simulink model "Yanwen_of_controller_mode"  (R2020a)
settings: Solver=FixedStepAuto  StartTime=0.0  StopTime=inf  FixedStep=SAMPLE_TIME  RelTol=1e-3
undefined symbols (not defined in the file or in its folder): D_saturation, DiscIntNeverNeededParam, G_correct_gain, GEAR_RATIO, I_saturation, MAX_QD, MAX_QDD, MAX_TAU, MJ_Test1_torque_mode, N, N_PLoop, N_VLoop, NUM_SEGMS, P_Kp, P_saturation, q_zero_offset, SAMPLE_TIME, theta_max, theta_min, v_des_saturation, V_Kd, V_Ki, V_Kp, v_threshold_I_stop
libraries: ighEthercatLib x38, simulink x9, simulink_extras x8, dspstat3 x3
(part 1 of 2)
settings Model: ExplicitPartitioning=on  Creator=86166  LastModifiedBy=win
settings OptimizationCC: EnhancedBackFolding=on  PassReuseOutputArgsThreshold=0  OptimizeBlockOrder=speed  DifferentSizesBufferReuse=on  OptimizationCustomize=off
settings DebuggingCC: ParameterTunabilityLossMsg=error
settings HardwareCC: ProdBitPerLong=64  ProdHWDeviceType=Intel->x86-64 (Linux 64)  TargetBitPerPointer=64  TargetBitPerSizeT=64  TargetBitPerPtrDiffT=64  TargetLongLongMode=on  TargetIntDivRoundTo=Zero  TargetEndianess=LittleEndian  TargetWordSize=64  TargetHWDeviceType=Custom Processor->MATLAB Host Computer  ProdEqTarget=off
settings RTWCC: Description=Generic Real-Time Target  SystemTargetFile=links_rtlnx_grt.tlc  GenCodeOnly=on  TemplateMakefile=links_rtlnx_grt.tmf  GenerateReport=on  RTWVerbose=off  CustomLibrary=libethercat.a  LaunchReport=on
settings CodeAppCC: ForceParamTrailComments=on  OperatorAnnotations=on
settings STFCustomTargetCC: ModelReferenceCompliant=off  CombineOutputUpdateFcns=on  SystemTargetFile=links_rtlnx_grt.tlc
settings GRTTargetCC: TargetLangStandard=C89/C90 (ANSI)  ModelReferenceCompliant=off  ParMdlRefBuildCompliant=off  CompOptLevelCompliant=off  ConcurrentExecutionCompliant=off  MatFileLogging=off  CPPClassGenCompliant=off  UseToolchainInfoCompliant=off  RTWCAPISignals=on  RTWCAPIParams=on  RTWCAPIRootIO=on

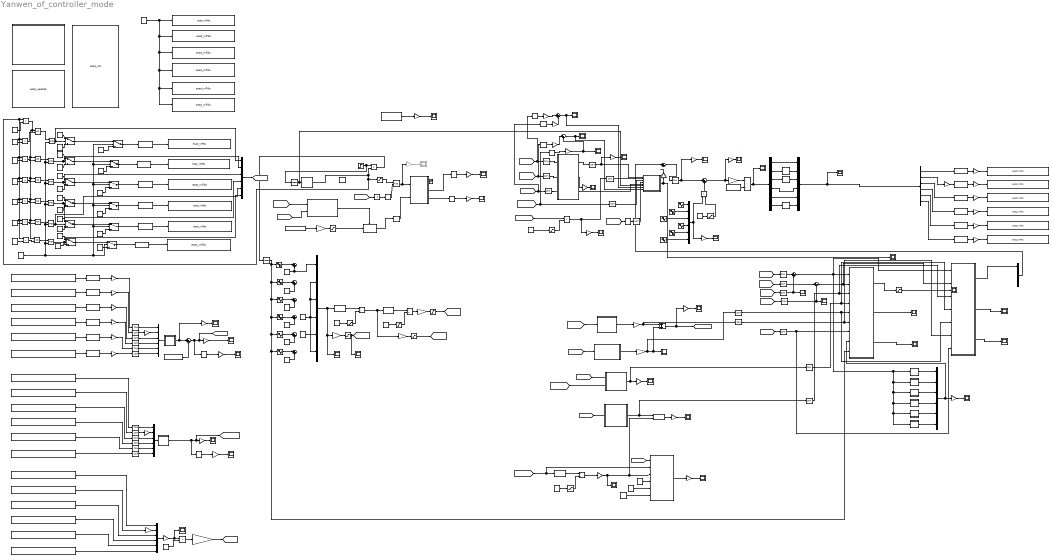
== system Yanwen_of_controller_mode ==
  note: 嵌套双环控制模块
  note: 8是位置模式，9是速度模式，10是力矩模式
  note: 关节使能之后才能启动轨迹规划
  note: 轨迹规划模块
  note: 编码器零位偏移量
  note: 模型识别变量模块
  note: 15是使能，6是去使能，128是驱动器初始化
  note: 连杆端的力矩值
  note: 使能控制
  note: 动力学模型计算模块
  note: 当前速度为零并且回到初始位置才能更新目标点
  note: 如果做数值仿真，则将阶跃信号替换sim_Step
  note: 模型初始化配置
  note: tau是连杆端力矩N.m，电机力矩输入单位是mN.m
  note: 所有的角度计算是基于弧度rad
  note: 滤波要用
  1dof_controller : MATLAB Function  TreatAsAtomicUnit=on
  Add2 : Sum
  C : Scope
  C_tau : Gain
  Compare To Zero : simulink/Logic and Bit Operations/Compare To Zero  relop=>  OutDataTypeStr=boolean
  Constant : Constant  Value=10
  Constant1 : Constant  Value=SAMPLE_TIME  SampleTime=SAMPLE_TIME
  Constant10 : Constant  Value=MJ_Test1_torque_mode
  Constant11 : Constant  Value=0
  Constant{12..13,17..21} (7 alike) : Constant  Value=6
  Constant{14..16,22..24} (6 alike) : Constant  Value=15
  Constant2 : Constant  Value=SAMPLE_TIME  SampleTime=SAMPLE_TIME
  Constant25 : Constant  Value=86  SampleTime=-1
  Constant26 : Constant  Value=4  SampleTime=-1
  Constant27 : Constant  Value=-5
  Constant28 : Constant  Value=10
  Constant29 : Constant  Value=0
  Constant3 : Constant  Value=0.001
  Constant30 : Constant  Value=90
  Constant33 : Constant  Value=SAMPLE_TIME  SampleTime=SAMPLE_TIME
  Constant{4..9} (6 alike) : Constant  Value=128
  Data Type Conversion{1,3..7,13..17,19} (12 alike) : DataTypeConversion  OutDataTypeStr=double
  Data Type Conversion{2,8..12} (6 alike) : DataTypeConversion  OutDataTypeStr=int32
  Demux : Demux  Outputs=6
  Demux2 : Demux  Outputs=6
  Difference : simulink/Discrete/Difference  ICPrevInput=zeros(1,6)  OutMin=[]  OutMax=[]  OutDataType=fixdt(1, 16)  OutScaling=2^-10  DoSatur=off
  Difference1 : simulink/Discrete/Difference  ICPrevInput=zeros(1,6)  OutMin=[]  OutMax=[]  OutDataType=fixdt(1, 16)  OutScaling=2^-10  DoSatur=off
  Difference2 : simulink/Discrete/Difference  ICPrevInput=zeros(1,6)  OutMin=[]  OutMax=[]  OutDataType=fixdt(1, 16)  OutScaling=2^-10  DoSatur=off
  Discrete-Time Integrator : DiscreteIntegrator  SampleTime=-1  ICPrevOutput=DiscIntNeverNeededParam  ICPrevScaledInput=DiscIntNeverNeededParam
  Discrete-Time Integrator1 : DiscreteIntegrator  SampleTime=-1  ICPrevOutput=DiscIntNeverNeededParam  ICPrevScaledInput=DiscIntNeverNeededParam
  Divide : Product  Inputs=*/  OutDataTypeStr=double
  Divide1 : Product  Inputs=*/
  Divide2 : Product  Inputs=*/
  Divide3 : Product  Inputs=*/
  Enabled Subsystem1 : Subsystem  TreatAsAtomicUnit=on
  G : Scope
  G_and_fric : Gain
  G_correct_gain : Gain  Gain=G_correct_gain
  Gain : Gain
  Gain{10..14,16} (6 alike) : Gain  OutDataTypeStr=Inherit: Same as input  ParamDataTypeStr=Inherit: Same as input
  JOINT2 Average1 : dspstat3/Moving Average  Method=Sliding window  ForgettingFactorPort=off  SpecifyWindowLength=on  WindowLength=2  ForgettingFactor=0.9  SimulateUsing=Code generation
  JOINT3 Average : dspstat3/Moving Average  Method=Sliding window  ForgettingFactorPort=off  SpecifyWindowLength=on  WindowLength=2  ForgettingFactor=0.9  SimulateUsing=Code generation
  JOINT3 Average1 : dspstat3/Moving Average  Method=Sliding window  ForgettingFactorPort=off  SpecifyWindowLength=on  WindowLength=3  ForgettingFactor=0.9  SimulateUsing=Code generation
  Kff_coef : Constant
  Logical Operator{,1..5} (6 alike) : Logic  Operator=OR  AllPortsSameDT=off  OutDataTypeStr=boolean
  Logical Operator{6..12} (7 alike) : Logic  AllPortsSameDT=off  OutDataTypeStr=boolean
  Logical Operator13 : Logic  Operator=NOT  AllPortsSameDT=off  OutDataTypeStr=boolean
  M*qdd : Gain
  M*qdd+C+G : Gain
  MJ_G_compen : MATLAB Function  TreatAsAtomicUnit=on  SystemSampleTime=SAMPLE_TIME
  MJ_M_matic : MATLAB Function  TreatAsAtomicUnit=on
  MJ_TAU : MATLAB Function  TreatAsAtomicUnit=on  SystemSampleTime=SAMPLE_TIME
  MJ_Traj2 : Subsystem
  MJ_V_compen : MATLAB Function  TreatAsAtomicUnit=on  SystemSampleTime=SAMPLE_TIME
  MJ_frict_compen1 : MATLAB Function  TreatAsAtomicUnit=on  SystemSampleTime=SAMPLE_TIME
  Memory : Memory  InitialCondition=zeros(1,6)  InheritSampleTime=on
  Memory1 : Memory  InitialCondition=[0, 0, 0, 0, 90, 0]  InheritSampleTime=on
  Model Source : Subsystem  mask(Model Source){ShowInLibBrowser=0}
      mask prompts: ShowInLibBrowser "Simulink:masks:CustCodeMaskParam1_MP"
      settings: CopyFcn=cccopyfcn(gcb)  OpenFcn=ccopenfcn('Model Source')
      mask Help: eval('feval(''rtwprivate'',''rtwhelpview'',''rtw_model_source_block'')');
      mask Display: disp('Model\nSource');
  Mux{,1..8} (9 alike) : Mux  Inputs=6
  PID_gain : Gain
  P_loop : Subsystem
  Product : Product  Multiplication=Matrix(*)
  Product{1..10} (10 alike) : Product
  Radians to Degrees{,1..7} (8 alike) : simulink_extras/Transformations/Radians to Degrees
  S-Function : ighEthercatLib/ecat_init  Priority=-100  icdFile=D:\RTLnxTest_Virtual\cooldriver_xpc.xml  domain_regs=|  pdo_entriesList=|  pdosList=|  slave_syncsList=|  vendor=1864  productCode=1  slaveCnt=6  dc=on  assign_activate=hex2dec('0x300')  sync0_cycle_time=1000000  sync0_shift_time=500000  sync1_cycle_time=0  sync1_shift_time=0  sampleTime=-1
      domain_regs=|
      | {{0,0,1864,1,0x6040,0,&g_processData[0]},
      | {0,0,1864,1,0x607a,0,&g_processData[1]},
      | {0,0,1864,1,0x60ff,0,&g_processData[2]},
      | {0,0,1864,1,0x6071,0,&g_processData[3]},
      | {0,0,1864,1,0x6060,0,&g_processData[4]},
      | {0,0,1864,1,0x5ffe,0,&g_processData[5]},
      | {0,0,1864,1,0x60b8,0,&g_processData[6]},
      | {0,0,1864,1,0x60b0,0,&g_processData[7]},
      | {0,0,1864,1,0x60b1,0,&g_processData[8]},
      | {0,0,1864,1,0x60b2,0,&g_processData[9]},
      | {0,0,1864,1,0x6041,0,&g_processData[10]},
      | {0,0,1864,1,0x6064,0,&g_processData[11]},
      | {0,0,1864,1,0x606c,0,&g_processData[12]},
      | {0,0,1864,1,0x6077,0,&g_processData[13]},
      | {0,0,1864,1,0x6061,0,&g_processData[14]},
      | {0,0,1864,1,0x5fff,0,&g_processData[15]},
      | {0,0,1864,1,0x60f4,0,&g_processData[16]},
      | {0,0,1864,1,0x60fd,0,&g_processData[17]},
      | {0,0,1864,1,0x60b9,0,&g_processData[18]},
      | {0,0,1864,1,0x60ba,0,&g_processData[19]},
      | {0,1,1864,1,0x6040,0,&g_processData[20]},
      | {0,1,1864,1,0x607a,0,&g_processData[21]},
      | {0,1,1864,1,0x60ff,0,&g_processData[22]},
      | {0,1,1864,1,0x6071,0,&g_processData[23]},
      | {0,1,1864,1,0x6060,0,&g_processData[24]},
      | {0,1,1864,1,0x5ffe,0,&g_processData[25]},
      | {0,1,1864,1,0x60b8,0,&g_processData[26]},
      | {0,1,1864,1,0x60b0,0,&g_processData[27]},
      | {0,1,1864,1,0x60b1,0,&g_processData[28]},
      | {0,1,1864,1,0x60b2,0,&g_processData[29]},
      | {0,1,1864,1,0x6041,0,&g_processData[30]},
      | {0,1,1864,1,0x6064,0,&g_processData[31]},
      | {0,1,1864,1,0x606c,0,&g_processData[32]},
      | {0,1,1864,1,0x6077,0,&g_processData[33]},
      | {0,1,1864,1,0x6061,0,&g_processData[34]},
      | {0,1,1864,1,0x5fff,0,&g_processData[35]},
      | {0,1,1864,1,0x60f4,0,&g_processData[36]},
      | {0,1,1864,1,0x60fd,0,&g_processData[37]},
      | {0,1,1864,1,0x60b9,0,&g_processData[38]},
      | {0,1,1864,1,0x60ba,0,&g_processData[39]},
      | {0,2,1864,1,0x6040,0,&g_processData[40]},
      | {0,2,1864,1,0x607a,0,&g_processData[41]},
      | {0,2,1864,1,0x60ff,0,&g_processData[42]},
      | {0,2,1864,1,0x6071,0,&g_processData[43]},
      | {0,2,1864,1,0x6060,0,&g_processData[44]},
      | {0,2,1864,1,0x5ffe,0,&g_processData[45]},
      | {0,2,1864,1,0x60b8,0,&g_processData[46]},
      | {0,2,1864,1,0x60b0,0,&g_processData[47]},
      | {0,2,1864,1,0x60b1,0,&g_processData[48]},
      | {0,2,1864,1,0x60b2,0,&g_processData[49]},
      | {0,2,1864,1,0x6041,0,&g_processData[50]},
      | {0,2,1864,1,0x6064,0,&g_processData[51]},
      | {0,2,1864,1,0x606c,0,&g_processData[52]},
      | {0,2,1864,1,0x6077,0,&g_processData[53]},
      | {0,2,1864,1,0x6061,0,&g_processData[54]},
      | {0,2,1864,1,0x5fff,0,&g_processData[55]},
      | {0,2,1864,1,0x60f4,0,&g_processData[56]},
      | {0,2,1864,1,0x60fd,0,&g_processData[57]},
      | {0,2,1864,1,0x60b9,0,&g_processData[58]},
      | {0,2,1864,1,0x60ba,0,&g_processData[59]},
      | {0,3,1864,1,0x6040,0,&g_processData[60]},
      | {0,3,1864,1,0x607a,0,&g_processData[61]},
      | {0,3,1864,1,0x60ff,0,&g_processData[62]},
      | {0,3,1864,1,0x6071,0,&g_processData[63]},
      | {0,3,1864,1,0x6060,0,&g_processData[64]},
      | {0,3,1864,1,0x5ffe,0,&g_processData[65]},
      | {0,3,1864,1,0x60b8,0,&g_processData[66]},
      | {0,3,1864,1,0x60b0,0,&g_processData[67]},
      | {0,3,1864,1,0x60b1,0,&g_processData[68]},
      | {0,3,1864,1,0x60b2,0,&g_processData[69]},
      | {0,3,1864,1,0x6041,0,&g_processData[70]},
      | {0,3,1864,1,0x6064,0,&g_processData[71]},
      | {0,3,1864,1,0x606c,0,&g_processData[72]},
      | {0,3,1864,1,0x6077,0,&g_processData[73]},
      | {0,3,1864,1,0x6061,0,&g_processData[74]},
      | {0,3,1864,1,0x5fff,0,&g_processData[75]},
      | {0,3,1864,1,0x60f4,0,&g_processData[76]},
      | {0,3,1864,1,0x60fd,0,&g_processData[77]},
      | {0,3,1864,1,0x60b9,0,&g_processData[78]},
      | {0,3,1864,1,0x60ba,0,&g_processData[79]},
      | {0,4,1864,1,0x6040,0,&g_processData[80]},
      | {0,4,1864,1,0x607a,0,&g_processData[81]},
      | {0,4,1864,1,0x60ff,0,&g_processData[82]},
      | {0,4,1864,1,0x6071,0,&g_processData[83]},
      | {0,4,1864,1,0x6060,0,&g_processData[84]},
      | {0,4,1864,1,0x5ffe,0,&g_processData[85]},
      | {0,4,1864,1,0x60b8,0,&g_processData[86]},
      | {0,4,1864,1,0x60b0,0,&g_processData[87]},
      | {0,4,1864,1,0x60b1,0,&g_processData[88]},
      | {0,4,1864,1,0x60b2,0,&g_processData[89]},
      | {0,4,1864,1,0x6041,0,&g_processData[90]},
      | {0,4,1864,1,0x6064,0,&g_processData[91]},
      | {0,4,1864,1,0x606c,0,&g_processData[92]},
      | {0,4,1864,1,0x6077,0,&g_processData[93]},
      | {0,4,1864,1,0x6061,0,&g_processData[94]},
      | {0,4,1864,1,0x5fff,0,&g_processData[95]},
      | {0,4,1864,1,0x60f4,0,&g_processData[96]},
      | {0,4,1864,1,0x60fd,0,&g_processData[97]},
      | {0,4,1864,1,0x60b9,0,&g_processData[98]},
      | {0,4,1864,1,0x60ba,0,&g_processData[99]},
      | {0,5,1864,1,0x6040,0,&g_processData[100]},
      | {0,5,1864,1,0x607a,0,&g_processData[101]},
      | {0,5,1864,1,0x60ff,0,&g_processData[102]},
      | {0,5,1864,1,0x6071,0,&g_processData[103]},
      | {0,5,1864,1,0x6060,0,&g_processData[104]},
      | {0,5,1864,1,0x5ffe,0,&g_processData[105]},
      | {0,5,1864,1,0x60b8,0,&g_processData[106]},
      | {0,5,1864,1,0x60b0,0,&g_processData[107]},
      | {0,5,1864,1,0x60b1,0,&g_processData[108]},
      | {0,5,1864,1,0x60b2,0,&g_processData[109]},
      | {0,5,1864,1,0x6041,0,&g_processData[110]},
      | {0,5,1864,1,0x6064,0,&g_processData[111]},
      | {0,5,1864,1,0x606c,0,&g_processData[112]},
      | {0,5,1864,1,0x6077,0,&g_processData[113]},
      | {0,5,1864,1,0x6061,0,&g_processData[114]},
      | {0,5,1864,1,0x5fff,0,&g_processData[115]},
      | {0,5,1864,1,0x60f4,0,&g_processData[116]},
      | {0,5,1864,1,0x60fd,0,&g_processData[117]},
      | {0,5,1864,1,0x60b9,0,&g_processData[118]},
      | {0,5,1864,1,0x60ba,0,&g_processData[119]},
      | }
      pdo_entriesList=|
      | {{{0x6040,0,16},/*Control Word*/
      | {0x607a,0,32},/*Target Position*/
      | {0x60ff,0,32},/*Target Velocity*/
      | {0x6071,0,16},/*Target Torque*/
      | {0x6060,0,8},/*Modes of operation*/
      | {0x5ffe,0,8},/*Dummy Byte*/
      | {0x60b8,0,16},/*Touch Probe Function*/
      | {0x60b0,0,32},/*Position Offset*/
      | {0x60b1,0,32},/*Velocity Offset*/
      | {0x60b2,0,16},/*Torque Offset*/
      | {0x6041,0,16},/*Status Word*/
      | {0x6064,0,32},/*Position Actual Value*/
      | {0x606c,0,32},/*Velocity Actual Value*/
      | {0x6077,0,16},/*Torque Actual Value*/
      | {0x6061,0,8},/*Mode of Operation Display*/
      | {0x5fff,0,8},/*Dummy Byte*/
      | {0x60f4,0,32},/*Following Error Actual Value*/
      | {0x60fd,0,32},/*Digital Inputs*/
      | {0x60b9,0,16},/*Touch Probe Status*/
      | {0x60ba,0,32},/*Touch Probe 1 Positive Edge Position Value*/
      | },{{0x6040,0,16},/*Control Word*/
      | {0x607a,0,32},/*Target Position*/
      | {0x60ff,0,32},/*Target Velocity*/
      | {0x6071,0,16},/*Target Torque*/
      | {0x6060,0,8},/*Modes of operation*/
      | {0x5ffe,0,8},/*Dummy Byte*/
      | {0x60b8,0,16},/*Touch Probe Function*/
      | {0x60b0,0,32},/*Position Offset*/
      | {0x60b1,0,32},/*Velocity Offset*/
      | {0x60b2,0,16},/*Torque Offset*/
      | {0x6041,0,16},/*Status Word*/
      | {0x6064,0,32},/*Position Actual Value*/
      | {0x606c,0,32},/*Velocity Actual Value*/
      | {0x6077,0,16},/*Torque Actual Value*/
      | {0x6061,0,8},/*Mode of Operation Display*/
      | {0x5fff,0,8},/*Dummy Byte*/
      | {0x60f4,0,32},/*Following Error Actual Value*/
      | {0x60fd,0,32},/*Digital Inputs*/
      | {0x60b9,0,16},/*Touch Probe Status*/
      | {0x60ba,0,32},/*Touch Probe 1 Positive Edge Position Value*/
      | },{{0x6040,0,16},/*Control Word*/
      | {0x607a,0,32},/*Target Position*/
      | {0x60ff,0,32},/*Target Velocity*/
      | {0x6071,0,16},/*Target Torque*/
      | {0x6060,0,8},/*Modes of operation*/
      | {0x5ffe,0,8},/*Dummy Byte*/
      | {0x60b8,0,16},/*Touch Probe Function*/
      | {0x60b0,0,32},/*Position Offset*/
      | {0x60b1,0,32},/*Velocity Offset*/
      | {0x60b2,0,16},/*Torque Offset*/
      | {0x6041,0,16},/*Status Word*/
      | {0x6064,0,32},/*Position Actual Value*/
      | {0x606c,0,32},/*Velocity Actual Value*/
      | {0x6077,0,16},/*Torque Actual Value*/
      | {0x6061,0,8},/*Mode of Operation Display*/
      | {0x5fff,0,8},/*Dummy Byte*/
      | {0x60f4,0,32},/*Following Error Actual Value*/
      | {0x60fd,0,32},/*Digital Inputs*/
      | {0x60b9,0,16},/*Touch Probe Status*/
      | {0x60ba,0,32},/*Touch Probe 1 Positive Edge Position Value*/
      | },{{0x6040,0,16},/*Control Word*/
      | {0x607a,0,32},/*Target Position*/
      | {0x60ff,0,32},/*Target Velocity*/
      | {0x6071,0,16},/*Target Torque*/
      | {0x6060,0,8},/*Modes of operation*/
      | {0x5ffe,0,8},/*Dummy Byte*/
      | {0x60b8,0,16},/*Touch Probe Function*/
      | {0x60b0,0,32},/*Position Offset*/
      | {0x60b1,0,32},/*Velocity Offset*/
      | {0x60b2,0,16},/*Torque Offset*/
      | {0x6041,0,16},/*Status Word*/
      | {0x6064,0,32},/*Position Actual Value*/
      | {0x606c,0,32},/*Velocity Actual Value*/
      | {0x6077,0,16},/*Torque Actual Value*/
      | {0x6061,0,8},/*Mode of Operation Display*/
      | {0x5fff,0,8},/*Dummy Byte*/
      | {0x60f4,0,32},/*Following Error Actual Value*/
      | {0x60fd,0,32},/*Digital Inputs*/
      | {0x60b9,0,16},/*Touch Probe Status*/
      | {0x60ba,0,32},/*Touch Probe 1 Positive Edge Position Value*/
      | },{{0x6040,0,16},/*Control Word*/
      | {0x607a,0,32},/*Target Position*/
      | {0x60ff,0,32},/*Target Velocity*/
      | {0x6071,0,16},/*Target Torque*/
      | {0x6060,0,8},/*Modes of operation*/
      | {0x5ffe,0,8},/*Dummy Byte*/
      | {0x60b8,0,16},/*Touch Probe Function*/
      | {0x60b0,0,32},/*Position Offset*/
      | {0x60b1,0,32},/*Velocity Offset*/
      | {0x60b2,0,16},/*Torque Offset*/
      | {0x6041,0,16},/*Status Word*/
      | {0x6064,0,32},/*Position Actual Value*/
      | {0x606c,0,32},/*Velocity Actual Value*/
      | {0x6077,0,16},/*Torque Actual Value*/
      | {0x6061,0,8},/*Mode of Operation Display*/
      | {0x5fff,0,8},/*Dummy Byte*/
      | {0x60f4,0,32},/*Following Error Actual Value*/
      | {0x60fd,0,32},/*Digital Inputs*/
      | {0x60b9,0,16},/*Touch Probe Status*/
      | {0x60ba,0,32},/*Touch Probe 1 Positive Edge Position Value*/
      | },{{0x6040,0,16},/*Control Word*/
      | {0x607a,0,32},/*Target Position*/
      | {0x60ff,0,32},/*Target Velocity*/
      | {0x6071,0,16},/*Target Torque*/
      | {0x6060,0,8},/*Modes of operation*/
      | {0x5ffe,0,8},/*Dummy Byte*/
      | {0x60b8,0,16},/*Touch Probe Function*/
      | {0x60b0,0,32},/*Position Offset*/
      | {0x60b1,0,32},/*Velocity Offset*/
      | {0x60b2,0,16},/*Torque Offset*/
      | {0x6041,0,16},/*Status Word*/
      | {0x6064,0,32},/*Position Actual Value*/
      | {0x606c,0,32},/*Velocity Actual Value*/
      | {0x6077,0,16},/*Torque Actual Value*/
      | {0x6061,0,8},/*Mode of Operation Display*/
      | {0x5fff,0,8},/*Dummy Byte*/
      | {0x60f4,0,32},/*Following Error Actual Value*/
      | {0x60fd,0,32},/*Digital Inputs*/
      | {0x60b9,0,16},/*Touch Probe Status*/
      | {0x60ba,0,32},/*Touch Probe 1 Positive Edge Position Value*/
      | }}
      pdosList=|
      | {{{0x1600,10,pdo_entries[0]+0},/*1st Receive PDO mapping*/
      | {0x1a00,10,pdo_entries[0]+10},/*1st Transmit PDO mapping*/
      | },{{0x1600,10,pdo_entries[1]+0},/*1st Receive PDO mapping*/
      | {0x1a00,10,pdo_entries[1]+10},/*1st Transmit PDO mapping*/
      | },{{0x1600,10,pdo_entries[2]+0},/*1st Receive PDO mapping*/
      | {0x1a00,10,pdo_entries[2]+10},/*1st Transmit PDO mapping*/
      | },{{0x1600,10,pdo_entries[3]+0},/*1st Receive PDO mapping*/
      | {0x1a00,10,pdo_entries[3]+10},/*1st Transmit PDO mapping*/
      | },{{0x1600,10,pdo_entries[4]+0},/*1st Receive PDO mapping*/
      | {0x1a00,10,pdo_entries[4]+10},/*1st Transmit PDO mapping*/
      | },{{0x1600,10,pdo_entries[5]+0},/*1st Receive PDO mapping*/
      | {0x1a00,10,pdo_entries[5]+10},/*1st Transmit PDO mapping*/
      | }}
      slave_syncsList=|
      | {{{0, EC_DIR_OUTPUT, 0, NULL, EC_WD_DISABLE},
      | {1, EC_DIR_INPUT, 0, NULL, EC_WD_DISABLE},
      | {2, EC_DIR_OUTPUT, 1, pdos[0] + 0, EC_WD_ENABLE},
      | {3, EC_DIR_INPUT, 1, pdos[0] + 1, EC_WD_DISABLE},
      | {0xff}},{{0, EC_DIR_OUTPUT, 0, NULL, EC_WD_DISABLE},
      | {1, EC_DIR_INPUT, 0, NULL, EC_WD_DISABLE},
      | {2, EC_DIR_OUTPUT, 1, pdos[1] + 0, EC_WD_ENABLE},
      | {3, EC_DIR_INPUT, 1, pdos[1] + 1, EC_WD_DISABLE},
      | {0xff}},{{0, EC_DIR_OUTPUT, 0, NULL, EC_WD_DISABLE},
      | {1, EC_DIR_INPUT, 0, NULL, EC_WD_DISABLE},
      | {2, EC_DIR_OUTPUT, 1, pdos[2] + 0, EC_WD_ENABLE},
      | {3, EC_DIR_INPUT, 1, pdos[2] + 1, EC_WD_DISABLE},
      | {0xff}},{{0, EC_DIR_OUTPUT, 0, NULL, EC_WD_DISABLE},
      | {1, EC_DIR_INPUT, 0, NULL, EC_WD_DISABLE},
      | {2, EC_DIR_OUTPUT, 1, pdos[3] + 0, EC_WD_ENABLE},
      | {3, EC_DIR_INPUT, 1, pdos[3] + 1, EC_WD_DISABLE},
      | {0xff}},{{0, EC_DIR_OUTPUT, 0, NULL, EC_WD_DISABLE},
      | {1, EC_DIR_INPUT, 0, NULL, EC_WD_DISABLE},
      | {2, EC_DIR_OUTPUT, 1, pdos[4] + 0, EC_WD_ENABLE},
      | {3, EC_DIR_INPUT, 1, pdos[4] + 1, EC_WD_DISABLE},
      | {0xff}},{{0, EC_DIR_OUTPUT, 0, NULL, EC_WD_DISABLE},
      | {1, EC_DIR_INPUT, 0, NULL, EC_WD_DISABLE},
      | {2, EC_DIR_OUTPUT, 1, pdos[5] + 0, EC_WD_ENABLE},
      | {3, EC_DIR_INPUT, 1, pdos[5] + 1, EC_WD_DISABLE},
      | {0xff}}}
  S-Function1 : ighEthercatLib/ecat_txPdo  Priority=0  f_name=Drive 6 (CoolDrive RC).1st Transmit PDO mapping.Velocity Actual Value  regDataTypes=[3 4 4 2 0 1 4 5 3 4 3 4 4 2 0 1 4 5 3 4 3 4 4 2 0 1 4 5 3 4 3 4 4 2 0 1 4 5 3 4 3 4 4 2 0 1 4 5 3 4 3 4 4 2 0 1 4 5 3 4]  PdoEntryIndex=[10 11 12 13 14 15 16 17 18 19 30 31 32 33 34 35 36 37 38 39 50 51 52 53 54 55 56 57 58 59 70 71 72 73 74 75 76 77 78 79 90 91 92 93 94 95 96 97 98 99 110 111 112 113 114 115 116 117 118 119]  pdoEntryName=Drive 6 (CoolDrive RC).1st Transmit PDO mapping.Velocity Actual Value  sampleTime=-1
  S-Function10 : ighEthercatLib/ecat_txPdo  Priority=0  f_name=Drive 4 (CoolDrive RC).1st Transmit PDO mapping.Velocity Actual Value  regDataTypes=[3 4 4 2 0 1 4 5 3 4 3 4 4 2 0 1 4 5 3 4 3 4 4 2 0 1 4 5 3 4 3 4 4 2 0 1 4 5 3 4 3 4 4 2 0 1 4 5 3 4 3 4 4 2 0 1 4 5 3 4]  PdoEntryIndex=[10 11 12 13 14 15 16 17 18 19 30 31 32 33 34 35 36 37 38 39 50 51 52 53 54 55 56 57 58 59 70 71 72 73 74 75 76 77 78 79 90 91 92 93 94 95 96 97 98 99 110 111 112 113 114 115 116 117 118 119]  pdoEntryName=Drive 4 (CoolDrive RC).1st Transmit PDO mapping.Velocity Actual Value  sampleTime=-1
  S-Function11 : ighEthercatLib/ecat_txPdo  Priority=0  f_name=Drive 3 (CoolDrive RC).1st Transmit PDO mapping.Velocity Actual Value  regDataTypes=[3 4 4 2 0 1 4 5 3 4 3 4 4 2 0 1 4 5 3 4 3 4 4 2 0 1 4 5 3 4 3 4 4 2 0 1 4 5 3 4 3 4 4 2 0 1 4 5 3 4 3 4 4 2 0 1 4 5 3 4]  PdoEntryIndex=[10 11 12 13 14 15 16 17 18 19 30 31 32 33 34 35 36 37 38 39 50 51 52 53 54 55 56 57 58 59 70 71 72 73 74 75 76 77 78 79 90 91 92 93 94 95 96 97 98 99 110 111 112 113 114 115 116 117 118 119]  pdoEntryName=Drive 3 (CoolDrive RC).1st Transmit PDO mapping.Velocity Actual Value  sampleTime=-1
  S-Function12 : ighEthercatLib/ecat_rxPdo  Priority=0  f_name=Drive 6 (CoolDrive RC).1st Receive PDO mapping.Target Torque  regDataTypes=[3 4 4 2 0 1 3 4 4 2 3 4 4 2 0 1 3 4 4 2 3 4 4 2 0 1 3 4 4 2 3 4 4 2 0 1 3 4 4 2 3 4 4 2 0 1 3 4 4 2 3 4 4 2 0 1 3 4 4 2]  PdoEntryIndex=[0 1 2 3 4 5 6 7 8 9 20 21 22 23 24 25 26 27 28 29 40 41 42 43 44 45 46 47 48 49 60 61 62 63 64 65 66 67 68 69 80 81 82 83 84 85 86 87 88 89 100 101 102 103 104 105 106 107 108 109]  pdoEntryName=Drive 6 (CoolDrive RC).1st Receive PDO mapping.Target Torque  sampleTime=-1
  S-Function13 : ighEthercatLib/ecat_txPdo  Priority=0  f_name=Drive 6 (CoolDrive RC).1st Transmit PDO mapping.Position Actual Value  regDataTypes=[3 4 4 2 0 1 4 5 3 4 3 4 4 2 0 1 4 5 3 4 3 4 4 2 0 1 4 5 3 4 3 4 4 2 0 1 4 5 3 4 3 4 4 2 0 1 4 5 3 4 3 4 4 2 0 1 4 5 3 4]  PdoEntryIndex=[10 11 12 13 14 15 16 17 18 19 30 31 32 33 34 35 36 37 38 39 50 51 52 53 54 55 56 57 58 59 70 71 72 73 74 75 76 77 78 79 90 91 92 93 94 95 96 97 98 99 110 111 112 113 114 115 116 117 118 119]  pdoEntryName=Drive 6 (CoolDrive RC).1st Transmit PDO mapping.Position Actual Value  sampleTime=-1
  S-Function14 : ighEthercatLib/ecat_rxPdo  Priority=0  f_name=Drive 5 (CoolDrive RC).1st Receive PDO mapping.Control Word  regDataTypes=[3 4 4 2 0 1 3 4 4 2 3 4 4 2 0 1 3 4 4 2 3 4 4 2 0 1 3 4 4 2 3 4 4 2 0 1 3 4 4 2 3 4 4 2 0 1 3 4 4 2 3 4 4 2 0 1 3 4 4 2]  PdoEntryIndex=[0 1 2 3 4 5 6 7 8 9 20 21 22 23 24 25 26 27 28 29 40 41 42 43 44 45 46 47 48 49 60 61 62 63 64 65 66 67 68 69 80 81 82 83 84 85 86 87 88 89 100 101 102 103 104 105 106 107 108 109]  pdoEntryName=Drive 5 (CoolDrive RC).1st Receive PDO mapping.Control Word  sampleTime=-1
  S-Function15 : ighEthercatLib/ecat_rxPdo  Priority=0  f_name=Drive 4 (CoolDrive RC).1st Receive PDO mapping.Control Word  regDataTypes=[3 4 4 2 0 1 3 4 4 2 3 4 4 2 0 1 3 4 4 2 3 4 4 2 0 1 3 4 4 2 3 4 4 2 0 1 3 4 4 2 3 4 4 2 0 1 3 4 4 2 3 4 4 2 0 1 3 4 4 2]  PdoEntryIndex=[0 1 2 3 4 5 6 7 8 9 20 21 22 23 24 25 26 27 28 29 40 41 42 43 44 45 46 47 48 49 60 61 62 63 64 65 66 67 68 69 80 81 82 83 84 85 86 87 88 89 100 101 102 103 104 105 106 107 108 109]  pdoEntryName=Drive 4 (CoolDrive RC).1st Receive PDO mapping.Control Word  sampleTime=-1
  S-Function16 : ighEthercatLib/ecat_rxPdo  Priority=0  f_name=Drive 3 (CoolDrive RC).1st Receive PDO mapping.Control Word  regDataTypes=[3 4 4 2 0 1 3 4 4 2 3 4 4 2 0 1 3 4 4 2 3 4 4 2 0 1 3 4 4 2 3 4 4 2 0 1 3 4 4 2 3 4 4 2 0 1 3 4 4 2 3 4 4 2 0 1 3 4 4 2]  PdoEntryIndex=[0 1 2 3 4 5 6 7 8 9 20 21 22 23 24 25 26 27 28 29 40 41 42 43 44 45 46 47 48 49 60 61 62 63 64 65 66 67 68 69 80 81 82 83 84 85 86 87 88 89 100 101 102 103 104 105 106 107 108 109]  pdoEntryName=Drive 3 (CoolDrive RC).1st Receive PDO mapping.Control Word  sampleTime=-1
  S-Function17 : ighEthercatLib/ecat_rxPdo  Priority=0  f_name=Drive 2 (CoolDrive RC).1st Receive PDO mapping.Control Word  regDataTypes=[3 4 4 2 0 1 3 4 4 2 3 4 4 2 0 1 3 4 4 2 3 4 4 2 0 1 3 4 4 2 3 4 4 2 0 1 3 4 4 2 3 4 4 2 0 1 3 4 4 2 3 4 4 2 0 1 3 4 4 2]  PdoEntryIndex=[0 1 2 3 4 5 6 7 8 9 20 21 22 23 24 25 26 27 28 29 40 41 42 43 44 45 46 47 48 49 60 61 62 63 64 65 66 67 68 69 80 81 82 83 84 85 86 87 88 89 100 101 102 103 104 105 106 107 108 109]  pdoEntryName=Drive 2 (CoolDrive RC).1st Receive PDO mapping.Control Word  sampleTime=-1
  S-Function18 : ighEthercatLib/ecat_rxPdo  Priority=0  f_name=Drive 1 (CoolDrive RC).1st Receive PDO mapping.Control Word  regDataTypes=[3 4 4 2 0 1 3 4 4 2 3 4 4 2 0 1 3 4 4 2 3 4 4 2 0 1 3 4 4 2 3 4 4 2 0 1 3 4 4 2 3 4 4 2 0 1 3 4 4 2 3 4 4 2 0 1 3 4 4 2]  PdoEntryIndex=[0 1 2 3 4 5 6 7 8 9 20 21 22 23 24 25 26 27 28 29 40 41 42 43 44 45 46 47 48 49 60 61 62 63 64 65 66 67 68 69 80 81 82 83 84 85 86 87 88 89 100 101 102 103 104 105 106 107 108 109]  pdoEntryName=Drive 1 (CoolDrive RC).1st Receive PDO mapping.Control Word  sampleTime=-1
  S-Function19 : ighEthercatLib/ecat_txPdo  Priority=0  f_name=Drive 5 (CoolDrive RC).1st Transmit PDO mapping.Position Actual Value  regDataTypes=[3 4 4 2 0 1 4 5 3 4 3 4 4 2 0 1 4 5 3 4 3 4 4 2 0 1 4 5 3 4 3 4 4 2 0 1 4 5 3 4 3 4 4 2 0 1 4 5 3 4 3 4 4 2 0 1 4 5 3 4]  PdoEntryIndex=[10 11 12 13 14 15 16 17 18 19 30 31 32 33 34 35 36 37 38 39 50 51 52 53 54 55 56 57 58 59 70 71 72 73 74 75 76 77 78 79 90 91 92 93 94 95 96 97 98 99 110 111 112 113 114 115 116 117 118 119]  pdoEntryName=Drive 5 (CoolDrive RC).1st Transmit PDO mapping.Position Actual Value  sampleTime=-1
  S-Function2 : ighEthercatLib/ecat_txPdo  Priority=0  f_name=Drive 5 (CoolDrive RC).1st Transmit PDO mapping.Velocity Actual Value  regDataTypes=[3 4 4 2 0 1 4 5 3 4 3 4 4 2 0 1 4 5 3 4 3 4 4 2 0 1 4 5 3 4 3 4 4 2 0 1 4 5 3 4 3 4 4 2 0 1 4 5 3 4 3 4 4 2 0 1 4 5 3 4]  PdoEntryIndex=[10 11 12 13 14 15 16 17 18 19 30 31 32 33 34 35 36 37 38 39 50 51 52 53 54 55 56 57 58 59 70 71 72 73 74 75 76 77 78 79 90 91 92 93 94 95 96 97 98 99 110 111 112 113 114 115 116 117 118 119]  pdoEntryName=Drive 5 (CoolDrive RC).1st Transmit PDO mapping.Velocity Actual Value  sampleTime=-1
  S-Function20 : ighEthercatLib/ecat_txPdo  Priority=0  f_name=Drive 4 (CoolDrive RC).1st Transmit PDO mapping.Position Actual Value  regDataTypes=[3 4 4 2 0 1 4 5 3 4 3 4 4 2 0 1 4 5 3 4 3 4 4 2 0 1 4 5 3 4 3 4 4 2 0 1 4 5 3 4 3 4 4 2 0 1 4 5 3 4 3 4 4 2 0 1 4 5 3 4]  PdoEntryIndex=[10 11 12 13 14 15 16 17 18 19 30 31 32 33 34 35 36 37 38 39 50 51 52 53 54 55 56 57 58 59 70 71 72 73 74 75 76 77 78 79 90 91 92 93 94 95 96 97 98 99 110 111 112 113 114 115 116 117 118 119]  pdoEntryName=Drive 4 (CoolDrive RC).1st Transmit PDO mapping.Position Actual Value  sampleTime=-1
  S-Function21 : ighEthercatLib/ecat_txPdo  Priority=0  f_name=Drive 3 (CoolDrive RC).1st Transmit PDO mapping.Position Actual Value  regDataTypes=[3 4 4 2 0 1 4 5 3 4 3 4 4 2 0 1 4 5 3 4 3 4 4 2 0 1 4 5 3 4 3 4 4 2 0 1 4 5 3 4 3 4 4 2 0 1 4 5 3 4 3 4 4 2 0 1 4 5 3 4]  PdoEntryIndex=[10 11 12 13 14 15 16 17 18 19 30 31 32 33 34 35 36 37 38 39 50 51 52 53 54 55 56 57 58 59 70 71 72 73 74 75 76 77 78 79 90 91 92 93 94 95 96 97 98 99 110 111 112 113 114 115 116 117 118 119]  pdoEntryName=Drive 3 (CoolDrive RC).1st Transmit PDO mapping.Position Actual Value  sampleTime=-1
  S-Function22 : ighEthercatLib/ecat_txPdo  Priority=0  f_name=Drive 2 (CoolDrive RC).1st Transmit PDO mapping.Position Actual Value  regDataTypes=[3 4 4 2 0 1 4 5 3 4 3 4 4 2 0 1 4 5 3 4 3 4 4 2 0 1 4 5 3 4 3 4 4 2 0 1 4 5 3 4 3 4 4 2 0 1 4 5 3 4 3 4 4 2 0 1 4 5 3 4]  PdoEntryIndex=[10 11 12 13 14 15 16 17 18 19 30 31 32 33 34 35 36 37 38 39 50 51 52 53 54 55 56 57 58 59 70 71 72 73 74 75 76 77 78 79 90 91 92 93 94 95 96 97 98 99 110 111 112 113 114 115 116 117 118 119]  pdoEntryName=Drive 2 (CoolDrive RC).1st Transmit PDO mapping.Position Actual Value  sampleTime=-1
  S-Function23 : ighEthercatLib/ecat_txPdo  Priority=0  f_name=Drive 1 (CoolDrive RC).1st Transmit PDO mapping.Position Actual Value  regDataTypes=[3 4 4 2 0 1 4 5 3 4 3 4 4 2 0 1 4 5 3 4 3 4 4 2 0 1 4 5 3 4 3 4 4 2 0 1 4 5 3 4 3 4 4 2 0 1 4 5 3 4 3 4 4 2 0 1 4 5 3 4]  PdoEntryIndex=[10 11 12 13 14 15 16 17 18 19 30 31 32 33 34 35 36 37 38 39 50 51 52 53 54 55 56 57 58 59 70 71 72 73 74 75 76 77 78 79 90 91 92 93 94 95 96 97 98 99 110 111 112 113 114 115 116 117 118 119]  pdoEntryName=Drive 1 (CoolDrive RC).1st Transmit PDO mapping.Position Actual Value  sampleTime=-1
  S-Function24 : ighEthercatLib/ecat_rxPdo  Priority=0  f_name=Drive 5 (CoolDrive RC).1st Receive PDO mapping.Target Torque  regDataTypes=[3 4 4 2 0 1 3 4 4 2 3 4 4 2 0 1 3 4 4 2 3 4 4 2 0 1 3 4 4 2 3 4 4 2 0 1 3 4 4 2 3 4 4 2 0 1 3 4 4 2 3 4 4 2 0 1 3 4 4 2]  PdoEntryIndex=[0 1 2 3 4 5 6 7 8 9 20 21 22 23 24 25 26 27 28 29 40 41 42 43 44 45 46 47 48 49 60 61 62 63 64 65 66 67 68 69 80 81 82 83 84 85 86 87 88 89 100 101 102 103 104 105 106 107 108 109]  pdoEntryName=Drive 5 (CoolDrive RC).1st Receive PDO mapping.Target Torque  sampleTime=-1
  S-Function25 : ighEthercatLib/ecat_rxPdo  Priority=0  f_name=Drive 4 (CoolDrive RC).1st Receive PDO mapping.Target Torque  regDataTypes=[3 4 4 2 0 1 3 4 4 2 3 4 4 2 0 1 3 4 4 2 3 4 4 2 0 1 3 4 4 2 3 4 4 2 0 1 3 4 4 2 3 4 4 2 0 1 3 4 4 2 3 4 4 2 0 1 3 4 4 2]  PdoEntryIndex=[0 1 2 3 4 5 6 7 8 9 20 21 22 23 24 25 26 27 28 29 40 41 42 43 44 45 46 47 48 49 60 61 62 63 64 65 66 67 68 69 80 81 82 83 84 85 86 87 88 89 100 101 102 103 104 105 106 107 108 109]  pdoEntryName=Drive 4 (CoolDrive RC).1st Receive PDO mapping.Target Torque  sampleTime=-1
  S-Function26 : ighEthercatLib/ecat_rxPdo  Priority=0  f_name=Drive 3 (CoolDrive RC).1st Receive PDO mapping.Target Torque  regDataTypes=[3 4 4 2 0 1 3 4 4 2 3 4 4 2 0 1 3 4 4 2 3 4 4 2 0 1 3 4 4 2 3 4 4 2 0 1 3 4 4 2 3 4 4 2 0 1 3 4 4 2 3 4 4 2 0 1 3 4 4 2]  PdoEntryIndex=[0 1 2 3 4 5 6 7 8 9 20 21 22 23 24 25 26 27 28 29 40 41 42 43 44 45 46 47 48 49 60 61 62 63 64 65 66 67 68 69 80 81 82 83 84 85 86 87 88 89 100 101 102 103 104 105 106 107 108 109]  pdoEntryName=Drive 3 (CoolDrive RC).1st Receive PDO mapping.Target Torque  sampleTime=-1
  S-Function27 : ighEthercatLib/ecat_rxPdo  Priority=0  f_name=Drive 2 (CoolDrive RC).1st Receive PDO mapping.Target Torque  regDataTypes=[3 4 4 2 0 1 3 4 4 2 3 4 4 2 0 1 3 4 4 2 3 4 4 2 0 1 3 4 4 2 3 4 4 2 0 1 3 4 4 2 3 4 4 2 0 1 3 4 4 2 3 4 4 2 0 1 3 4 4 2]  PdoEntryIndex=[0 1 2 3 4 5 6 7 8 9 20 21 22 23 24 25 26 27 28 29 40 41 42 43 44 45 46 47 48 49 60 61 62 63 64 65 66 67 68 69 80 81 82 83 84 85 86 87 88 89 100 101 102 103 104 105 106 107 108 109]  pdoEntryName=Drive 2 (CoolDrive RC).1st Receive PDO mapping.Target Torque  sampleTime=-1
  S-Function28 : ighEthercatLib/ecat_rxPdo  Priority=0  f_name=Drive 1 (CoolDrive RC).1st Receive PDO mapping.Target Torque  regDataTypes=[3 4 4 2 0 1 3 4 4 2 3 4 4 2 0 1 3 4 4 2 3 4 4 2 0 1 3 4 4 2 3 4 4 2 0 1 3 4 4 2 3 4 4 2 0 1 3 4 4 2 3 4 4 2 0 1 3 4 4 2]  PdoEntryIndex=[0 1 2 3 4 5 6 7 8 9 20 21 22 23 24 25 26 27 28 29 40 41 42 43 44 45 46 47 48 49 60 61 62 63 64 65 66 67 68 69 80 81 82 83 84 85 86 87 88 89 100 101 102 103 104 105 106 107 108 109]  pdoEntryName=Drive 1 (CoolDrive RC).1st Receive PDO mapping.Target Torque  sampleTime=-1
  S-Function29 : ighEthercatLib/ecat_txPdo  Priority=0  f_name=Drive 2 (CoolDrive RC).1st Transmit PDO mapping.Velocity Actual Value  regDataTypes=[3 4 4 2 0 1 4 5 3 4 3 4 4 2 0 1 4 5 3 4 3 4 4 2 0 1 4 5 3 4 3 4 4 2 0 1 4 5 3 4 3 4 4 2 0 1 4 5 3 4 3 4 4 2 0 1 4 5 3 4]  PdoEntryIndex=[10 11 12 13 14 15 16 17 18 19 30 31 32 33 34 35 36 37 38 39 50 51 52 53 54 55 56 57 58 59 70 71 72 73 74 75 76 77 78 79 90 91 92 93 94 95 96 97 98 99 110 111 112 113 114 115 116 117 118 119]  pdoEntryName=Drive 2 (CoolDrive RC).1st Transmit PDO mapping.Velocity Actual Value  sampleTime=-1
  S-Function3 : ighEthercatLib/ecat_rxPdo  Priority=0  f_name=Drive 1 (CoolDrive RC).1st Receive PDO mapping.Modes of operation  regDataTypes=[3 4 4 2 0 1 3 4 4 2 3 4 4 2 0 1 3 4 4 2 3 4 4 2 0 1 3 4 4 2 3 4 4 2 0 1 3 4 4 2 3 4 4 2 0 1 3 4 4 2 3 4 4 2 0 1 3 4 4 2]  PdoEntryIndex=[0 1 2 3 4 5 6 7 8 9 20 21 22 23 24 25 26 27 28 29 40 41 42 43 44 45 46 47 48 49 60 61 62 63 64 65 66 67 68 69 80 81 82 83 84 85 86 87 88 89 100 101 102 103 104 105 106 107 108 109]  pdoEntryName=Drive 1 (CoolDrive RC).1st Receive PDO mapping.Modes of operation  sampleTime=-1
  S-Function30 : ighEthercatLib/ecat_txPdo  Priority=0  f_name=Drive 1 (CoolDrive RC).1st Transmit PDO mapping.Velocity Actual Value  regDataTypes=[3 4 4 2 0 1 4 5 3 4 3 4 4 2 0 1 4 5 3 4 3 4 4 2 0 1 4 5 3 4 3 4 4 2 0 1 4 5 3 4 3 4 4 2 0 1 4 5 3 4 3 4 4 2 0 1 4 5 3 4]  PdoEntryIndex=[10 11 12 13 14 15 16 17 18 19 30 31 32 33 34 35 36 37 38 39 50 51 52 53 54 55 56 57 58 59 70 71 72 73 74 75 76 77 78 79 90 91 92 93 94 95 96 97 98 99 110 111 112 113 114 115 116 117 118 119]  pdoEntryName=Drive 1 (CoolDrive RC).1st Transmit PDO mapping.Velocity Actual Value  sampleTime=-1
  S-Function31 : ighEthercatLib/ecat_txPdo  Priority=0  f_name=Drive 6 (CoolDrive RC).1st Transmit PDO mapping.Torque Actual Value  regDataTypes=[3 4 4 2 0 1 4 5 3 4 3 4 4 2 0 1 4 5 3 4 3 4 4 2 0 1 4 5 3 4 3 4 4 2 0 1 4 5 3 4 3 4 4 2 0 1 4 5 3 4 3 4 4 2 0 1 4 5 3 4]  PdoEntryIndex=[10 11 12 13 14 15 16 17 18 19 30 31 32 33 34 35 36 37 38 39 50 51 52 53 54 55 56 57 58 59 70 71 72 73 74 75 76 77 78 79 90 91 92 93 94 95 96 97 98 99 110 111 112 113 114 115 116 117 118 119]  pdoEntryName=Drive 6 (CoolDrive RC).1st Transmit PDO mapping.Torque Actual Value  sampleTime=-1
  S-Function32 : ighEthercatLib/ecat_txPdo  Priority=0  f_name=Drive 4 (CoolDrive RC).1st Transmit PDO mapping.Torque Actual Value  regDataTypes=[3 4 4 2 0 1 4 5 3 4 3 4 4 2 0 1 4 5 3 4 3 4 4 2 0 1 4 5 3 4 3 4 4 2 0 1 4 5 3 4 3 4 4 2 0 1 4 5 3 4 3 4 4 2 0 1 4 5 3 4]  PdoEntryIndex=[10 11 12 13 14 15 16 17 18 19 30 31 32 33 34 35 36 37 38 39 50 51 52 53 54 55 56 57 58 59 70 71 72 73 74 75 76 77 78 79 90 91 92 93 94 95 96 97 98 99 110 111 112 113 114 115 116 117 118 119]  pdoEntryName=Drive 4 (CoolDrive RC).1st Transmit PDO mapping.Torque Actual Value  sampleTime=-1
  S-Function33 : ighEthercatLib/ecat_txPdo  Priority=0  f_name=Drive 3 (CoolDrive RC).1st Transmit PDO mapping.Torque Actual Value  regDataTypes=[3 4 4 2 0 1 4 5 3 4 3 4 4 2 0 1 4 5 3 4 3 4 4 2 0 1 4 5 3 4 3 4 4 2 0 1 4 5 3 4 3 4 4 2 0 1 4 5 3 4 3 4 4 2 0 1 4 5 3 4]  PdoEntryIndex=[10 11 12 13 14 15 16 17 18 19 30 31 32 33 34 35 36 37 38 39 50 51 52 53 54 55 56 57 58 59 70 71 72 73 74 75 76 77 78 79 90 91 92 93 94 95 96 97 98 99 110 111 112 113 114 115 116 117 118 119]  pdoEntryName=Drive 3 (CoolDrive RC).1st Transmit PDO mapping.Torque Actual Value  sampleTime=-1
  S-Function34 : ighEthercatLib/ecat_txPdo  Priority=0  f_name=Drive 5 (CoolDrive RC).1st Transmit PDO mapping.Torque Actual Value  regDataTypes=[3 4 4 2 0 1 4 5 3 4 3 4 4 2 0 1 4 5 3 4 3 4 4 2 0 1 4 5 3 4 3 4 4 2 0 1 4 5 3 4 3 4 4 2 0 1 4 5 3 4 3 4 4 2 0 1 4 5 3 4]  PdoEntryIndex=[10 11 12 13 14 15 16 17 18 19 30 31 32 33 34 35 36 37 38 39 50 51 52 53 54 55 56 57 58 59 70 71 72 73 74 75 76 77 78 79 90 91 92 93 94 95 96 97 98 99 110 111 112 113 114 115 116 117 118 119]  pdoEntryName=Drive 5 (CoolDrive RC).1st Transmit PDO mapping.Torque Actual Value  sampleTime=-1
  S-Function35 : ighEthercatLib/ecat_txPdo  Priority=0  f_name=Drive 2 (CoolDrive RC).1st Transmit PDO mapping.Torque Actual Value  regDataTypes=[3 4 4 2 0 1 4 5 3 4 3 4 4 2 0 1 4 5 3 4 3 4 4 2 0 1 4 5 3 4 3 4 4 2 0 1 4 5 3 4 3 4 4 2 0 1 4 5 3 4 3 4 4 2 0 1 4 5 3 4]  PdoEntryIndex=[10 11 12 13 14 15 16 17 18 19 30 31 32 33 34 35 36 37 38 39 50 51 52 53 54 55 56 57 58 59 70 71 72 73 74 75 76 77 78 79 90 91 92 93 94 95 96 97 98 99 110 111 112 113 114 115 116 117 118 119]  pdoEntryName=Drive 2 (CoolDrive RC).1st Transmit PDO mapping.Torque Actual Value  sampleTime=-1
  S-Function36 : ighEthercatLib/ecat_txPdo  Priority=0  f_name=Drive 1 (CoolDrive RC).1st Transmit PDO mapping.Torque Actual Value  regDataTypes=[3 4 4 2 0 1 4 5 3 4 3 4 4 2 0 1 4 5 3 4 3 4 4 2 0 1 4 5 3 4 3 4 4 2 0 1 4 5 3 4 3 4 4 2 0 1 4 5 3 4 3 4 4 2 0 1 4 5 3 4]  PdoEntryIndex=[10 11 12 13 14 15 16 17 18 19 30 31 32 33 34 35 36 37 38 39 50 51 52 53 54 55 56 57 58 59 70 71 72 73 74 75 76 77 78 79 90 91 92 93 94 95 96 97 98 99 110 111 112 113 114 115 116 117 118 119]  pdoEntryName=Drive 1 (CoolDrive RC).1st Transmit PDO mapping.Torque Actual Value  sampleTime=-1
  S-Function4 : ighEthercatLib/ecat_rxPdo  Priority=0  f_name=Drive 2 (CoolDrive RC).1st Receive PDO mapping.Modes of operation  regDataTypes=[3 4 4 2 0 1 3 4 4 2 3 4 4 2 0 1 3 4 4 2 3 4 4 2 0 1 3 4 4 2 3 4 4 2 0 1 3 4 4 2 3 4 4 2 0 1 3 4 4 2 3 4 4 2 0 1 3 4 4 2]  PdoEntryIndex=[0 1 2 3 4 5 6 7 8 9 20 21 22 23 24 25 26 27 28 29 40 41 42 43 44 45 46 47 48 49 60 61 62 63 64 65 66 67 68 69 80 81 82 83 84 85 86 87 88 89 100 101 102 103 104 105 106 107 108 109]  pdoEntryName=Drive 2 (CoolDrive RC).1st Receive PDO mapping.Modes of operation  sampleTime=-1
  S-Function5 : ighEthercatLib/ecat_rxPdo  Priority=0  f_name=Drive 3 (CoolDrive RC).1st Receive PDO mapping.Modes of operation  regDataTypes=[3 4 4 2 0 1 3 4 4 2 3 4 4 2 0 1 3 4 4 2 3 4 4 2 0 1 3 4 4 2 3 4 4 2 0 1 3 4 4 2 3 4 4 2 0 1 3 4 4 2 3 4 4 2 0 1 3 4 4 2]  PdoEntryIndex=[0 1 2 3 4 5 6 7 8 9 20 21 22 23 24 25 26 27 28 29 40 41 42 43 44 45 46 47 48 49 60 61 62 63 64 65 66 67 68 69 80 81 82 83 84 85 86 87 88 89 100 101 102 103 104 105 106 107 108 109]  pdoEntryName=Drive 3 (CoolDrive RC).1st Receive PDO mapping.Modes of operation  sampleTime=-1
  S-Function6 : ighEthercatLib/ecat_rxPdo  Priority=0  f_name=Drive 4 (CoolDrive RC).1st Receive PDO mapping.Modes of operation  regDataTypes=[3 4 4 2 0 1 3 4 4 2 3 4 4 2 0 1 3 4 4 2 3 4 4 2 0 1 3 4 4 2 3 4 4 2 0 1 3 4 4 2 3 4 4 2 0 1 3 4 4 2 3 4 4 2 0 1 3 4 4 2]  PdoEntryIndex=[0 1 2 3 4 5 6 7 8 9 20 21 22 23 24 25 26 27 28 29 40 41 42 43 44 45 46 47 48 49 60 61 62 63 64 65 66 67 68 69 80 81 82 83 84 85 86 87 88 89 100 101 102 103 104 105 106 107 108 109]  pdoEntryName=Drive 4 (CoolDrive RC).1st Receive PDO mapping.Modes of operation  sampleTime=-1
  S-Function7 : ighEthercatLib/ecat_rxPdo  Priority=0  f_name=Drive 5 (CoolDrive RC).1st Receive PDO mapping.Modes of operation  regDataTypes=[3 4 4 2 0 1 3 4 4 2 3 4 4 2 0 1 3 4 4 2 3 4 4 2 0 1 3 4 4 2 3 4 4 2 0 1 3 4 4 2 3 4 4 2 0 1 3 4 4 2 3 4 4 2 0 1 3 4 4 2]  PdoEntryIndex=[0 1 2 3 4 5 6 7 8 9 20 21 22 23 24 25 26 27 28 29 40 41 42 43 44 45 46 47 48 49 60 61 62 63 64 65 66 67 68 69 80 81 82 83 84 85 86 87 88 89 100 101 102 103 104 105 106 107 108 109]  pdoEntryName=Drive 5 (CoolDrive RC).1st Receive PDO mapping.Modes of operation  sampleTime=-1
  S-Function8 : ighEthercatLib/ecat_rxPdo  Priority=0  f_name=Drive 6 (CoolDrive RC).1st Receive PDO mapping.Modes of operation  regDataTypes=[3 4 4 2 0 1 3 4 4 2 3 4 4 2 0 1 3 4 4 2 3 4 4 2 0 1 3 4 4 2 3 4 4 2 0 1 3 4 4 2 3 4 4 2 0 1 3 4 4 2 3 4 4 2 0 1 3 4 4 2]  PdoEntryIndex=[0 1 2 3 4 5 6 7 8 9 20 21 22 23 24 25 26 27 28 29 40 41 42 43 44 45 46 47 48 49 60 61 62 63 64 65 66 67 68 69 80 81 82 83 84 85 86 87 88 89 100 101 102 103 104 105 106 107 108 109]  pdoEntryName=Drive 6 (CoolDrive RC).1st Receive PDO mapping.Modes of operation  sampleTime=-1
  S-Function9 : ighEthercatLib/ecat_rxPdo  Priority=0  f_name=Drive 6 (CoolDrive RC).1st Receive PDO mapping.Control Word  regDataTypes=[3 4 4 2 0 1 3 4 4 2 3 4 4 2 0 1 3 4 4 2 3 4 4 2 0 1 3 4 4 2 3 4 4 2 0 1 3 4 4 2 3 4 4 2 0 1 3 4 4 2 3 4 4 2 0 1 3 4 4 2]  PdoEntryIndex=[0 1 2 3 4 5 6 7 8 9 20 21 22 23 24 25 26 27 28 29 40 41 42 43 44 45 46 47 48 49 60 61 62 63 64 65 66 67 68 69 80 81 82 83 84 85 86 87 88 89 100 101 102 103 104 105 106 107 108 109]  pdoEntryName=Drive 6 (CoolDrive RC).1st Receive PDO mapping.Control Word  sampleTime=-1
  Saturation{,5..6,8} (4 alike) : Saturate  UpperLimit=theta_max  LowerLimit=theta_min
  Saturation1 : Saturate  UpperLimit=1  LowerLimit=1.0e-5
  Saturation10 : Saturate  UpperLimit=200  LowerLimit=-200
  Saturation2 : Saturate  UpperLimit=1  LowerLimit=0
  Saturation3 : Saturate  UpperLimit=1  LowerLimit=0
  Saturation4 : Saturate  UpperLimit=1  LowerLimit=0
  Saturation7 : Saturate  UpperLimit=1  LowerLimit=1.0e-5
  Saturation9 : Saturate  UpperLimit=1  LowerLimit=1.0e-5
  Scope{,1..2,4..31} (31 alike) : Scope
  Scope3 : Scope  Commented=on
  Sine Wave Function : Sin  TimeSource=Use external signal  Amplitude=5  Frequency=0.2  SampleTime=0
  Sine Wave Function1 : Sin  TimeSource=Use external signal  Amplitude=2  Frequency=0.2  SampleTime=0
  Sine Wave Function2 : Sin  TimeSource=Use external signal  Amplitude=-2  Frequency=0.2  SampleTime=0
  Sine Wave Function3 : Sin  TimeSource=Use external signal  Amplitude=5  Frequency=0.2  SampleTime=0
  Sine Wave Function4 : Sin  TimeSource=Use external signal  Amplitude=4  Frequency=0.2  Phase=pi/2  SampleTime=0
  Sine Wave Function5 : Sin  TimeSource=Use external signal  Amplitude=-2  Frequency=0.2  Phase=pi/2  SampleTime=0
  Subsystem6 : Subsystem
  Sum{,3,6..7,9..12} (8 alike) : Sum  Inputs=|++
  Sum of Elements : Sum  Inputs=+
  Sum{1..2,4..5,8} (5 alike) : Sum  Inputs=|+-
  Switch{,1..5} (6 alike) : Switch  Criteria=u2 > Threshold  Threshold=0.5
  Switch{6..11} (6 alike) : Switch  Criteria=u2 > Threshold
  Terminator : Terminator
  V_loop : Subsystem
  V_out{,1..4} (5 alike) : Gain
  Zero-Order Hold{,13..15,24..27} (8 alike) : ZeroOrderHold  SampleTime=SAMPLE_TIME*N_VLoop
  Zero-Order Hold{1..12} (12 alike) : ZeroOrderHold  SampleTime=-1
  Zero-Order Hold{16..23} (8 alike) : ZeroOrderHold  SampleTime=SAMPLE_TIME*N_PLoop
  atual_raw_tau : Scope
  atual_tau : Product  OutDataTypeStr=double
  atual_tau_rod : Gain  Gain=GEAR_RATIO
  controller1 : MATLAB Function  TreatAsAtomicUnit=on
  degree2rad{,1..3} (4 alike) : Gain  Gain=pi/180
  dingshichufa : MATLAB Function  TreatAsAtomicUnit=on
  disturb_{1..6} (6 alike) : Sin  Amplitude=0.1  SampleTime=SAMPLE_TIME
  disturb_gain : Constant  Value=0
  ecat_update : ighEthercatLib/ecat_update  Priority=1  SampleTime=-1
  enable1 : Constant  Value=0  OutDataTypeStr=double
  enable{2..6} (5 alike) : Constant  Value=0
  enable_all : Constant  Value=0  OutDataTypeStr=double
  err : Gain
  f_ext : Constant  Value=[0, 0, 0]
  feed_forward_tau : Scope
  fri_gain : Gain
  fuzzy_logic_system1 : MATLAB Function  TreatAsAtomicUnit=on
  fuzzy_logic_system2 : MATLAB Function  TreatAsAtomicUnit=on
  fuzzy_logic_system3 : MATLAB Function  TreatAsAtomicUnit=on
  fuzzy_logic_system4 : MATLAB Function  TreatAsAtomicUnit=on
  fuzzy_logic_system5 : MATLAB Function  TreatAsAtomicUnit=on
  fuzzy_logic_system6 : MATLAB Function  TreatAsAtomicUnit=on
  gear_ratio1 : Constant  Value=GEAR_RATIO  OutDataTypeStr=double
  get_tau : Gain  OutDataTypeStr=double
  grav : Constant  Value=[0, 0, 9.81]
  inc2rad : Subsystem
  inc2rad1 : Subsystem
  init_clear : Constant  Value=0
  joint2_inver_dir1 : Gain  Gain=-1  OutDataTypeStr=Inherit: Same as input  ParamDataTypeStr=Inherit: Same as input
  joint2_inver_dir2 : Gain  Gain=-1  OutDataTypeStr=Inherit: Same as input  ParamDataTypeStr=Inherit: Same as input
  joint2_inver_dir3 : Gain  Gain=-1  OutDataTypeStr=Inherit: Same as input
  joint2_inver_dir4 : Gain  Gain=-1  OutDataTypeStr=Inherit: Same as input
  k : Gain  Gain=1000  ParamDataTypeStr=int32
  n_ext : Constant  Value=[0, 0, 0]
  offset_q : Constant  Value=q_zero_offset
  pos1 : Gain  OutDataTypeStr=Inherit: Same as input
  pos{2..6} (5 alike) : Gain  OutDataTypeStr=Inherit: Same as input  ParamDataTypeStr=Inherit: Same as input
  q_degree : Gain  OutDataTypeStr=Inherit: Same as input  ParamDataTypeStr=Inherit: Same as input
  q_des_degree : Constant  Value=[0, 0, 0, 0, 90, 0]
  q_des_t : Gain
  q_rad : Gain  OutDataTypeStr=Inherit: Same as input  ParamDataTypeStr=Inherit: Same as input
  q_rad_raw : Gain  OutDataTypeStr=Inherit: Same as input  ParamDataTypeStr=Inherit: Same as input
  qd_degree : Gain  OutDataTypeStr=Inherit: Same as input
  qd_des_t : Gain
  qd_rad : Gain  OutDataTypeStr=Inherit: Same as input
  qdd : Gain
  qdd1 : Gain
  qdd_atual : Scope
  sim_Step : Step  Time=2
  start : Gain  Commented=on
  tau_all : Scope
  tau_disturb : Gain
  tau_ff : Gain
  tau_final : Gain
  tau_out : Gain
  traj_enable : Constant  Value=0
  wires:
  Logical Operator11/1 -> Switch7/2, Mux3/1
  Radians to Degrees/1 -> q_degree/1
  qd_rad/1 -> Scope4/1  "qd_actual"
  Radians to Degrees2/1 -> qd_degree/1
  Zero-Order Hold2/1 -> joint2_inver_dir4/1
  Constant9/1 -> Switch5/3
  Switch4/1 -> Data Type Conversion13/1
  Constant5/1 -> Switch1/3
  Logical Operator8/1 -> Mux3/4, Switch10/2
  Logical Operator9/1 -> Mux3/3, Switch9/2
  Switch3/1 -> Data Type Conversion14/1
  Zero-Order Hold3/1 -> Mux2/3
  pos1/1 -> S-Function28/1  "actuastatus1"
  Data Type Conversion14/1 -> S-Function16/1
  Demux/1 -> Data Type Conversion7/1
  S-Function11/1 -> Zero-Order Hold3/1
  Demux/5 -> Data Type Conversion3/1
  Switch5/1 -> Data Type Conversion19/1
  Gain11/1 -> Zero-Order Hold11/1  "Encode5"
  Demux/3 -> Data Type Conversion5/1
  Gain12/1 -> Zero-Order Hold10/1  "Encode4"
  pos6/1 -> S-Function12/1  "actuastatus6"
  Gain10/1 -> Zero-Order Hold12/1  "Encode6"
  dingshichufa/1(trajflag) -> Product9/1, Product8/1, Product7/1, Product6/1, Product4/1, Product10/1, Product5/1, Saturation2/1, Product3/2
  Logical Operator7/1 -> Switch11/2, Mux3/5
  q_rad/1 -> Scope15/1  "q_actual"
  Data Type Conversion15/1 -> S-Function15/1
  Gain13/1 -> Zero-Order Hold9/1  "Encode3"
  Sum2/1 -> [q_actual], q_rad/1, Radians to Degrees/1
  q_rad_raw/1 -> Scope17/1
  Zero-Order Hold11/1 -> Mux/5
  Zero-Order Hold12/1 -> Mux/6
  Data Type Conversion13/1 -> S-Function17/1
  gear_ratio1/1 -> Divide/2
  S-Function29/1 -> Zero-Order Hold2/1
  Memory/1 -> Logical Operator13/1
  err/1 -> Scope9/1
  grav/1 -> MJ_TAU/6(grav)
  qdd/1 -> MJ_TAU/3(qdd), Product/2, qdd_atual/1  "qdd_actual"
  Data Type Conversion12/1 -> Gain16/1
  disturb_1/1 -> Mux6/1
  atual_tau/1 -> atual_tau_rod/1
  [qd_actual] -> MJ_V_compen/2(qd)
  Constant20/1 -> Switch8/3
  [q_actual] -> Radians to Degrees7/1, Zero-Order Hold19/1
  Sum/1 -> tau_final/1, k/1
  degree2rad/1 -> Saturation/1
  k/1 -> Divide/1
  Logical Operator10/1 -> Mux3/2, Switch8/2
  Data Type Conversion7/1 -> pos1/1
  Zero-Order Hold/1 -> V_loop/3(actual_qd)
  init_clear/1 -> Switch/2, Switch5/2, Switch4/2, Switch3/2, Switch2/2, Switch1/2, Logical Operator6/2, Logical Operator11/2, Logical Operator10/2, Logical Operator9/2, Logical Operator8/2, Logical Operator7/2
  S-Function21/1 -> Data Type Conversion10/1
  Radians to Degrees1/1 -> q_des_t/1
  [q_actual] -> MJ_TAU/1(q)
  Mux2/1 -> inc2rad1/1(inc)
  Saturation2/1 -> Logical Operator12/1
  Constant24/1 -> Switch9/1
  Demux/2 -> joint2_inver_dir2/1
  Saturation1/1 -> Divide1/2
  Demux/4 -> Data Type Conversion4/1
  Mux1/1 -> get_tau/1
  Constant8/1 -> Switch4/3
  inc2rad/1(rad) -> q_rad_raw/1, Sum2/1
  [q_des] -> Subsystem6/1(q_traj_rad)
  [q_des] -> Radians to Degrees6/1, Zero-Order Hold16/1
  S-Function30/1 -> Zero-Order Hold1/1
  [feedforward_tau] -> Product1/1
  MJ_Traj2/1(dt) -> Terminator/1
  MJ_TAU/1(ALL_tau) -> M*qdd+C+G/1
  tau_final/1 -> Scope12/1  "tau_final"
  Demux2/3 -> JOINT3 Average/1
  Zero-Order Hold8/1 -> joint2_inver_dir1/1
  Constant4/1 -> Switch/3
  Sum of Elements/1 -> Compare To Zero/1
  Zero-Order Hold4/1 -> Mux2/4
  Zero-Order Hold16/1 -> P_loop/1(q_des)
  M*qdd/1 -> Scope7/1
  Product1/1 -> tau_ff/1, Zero-Order Hold14/1
  Demux2/6 -> JOINT3 Average1/1
  Logical Operator4/1 -> Logical Operator7/1
  Zero-Order Hold7/1 -> Mux/1
  Switch2/1 -> Data Type Conversion15/1
  Zero-Order Hold5/1 -> Mux2/5
  Data Type Conversion5/1 -> pos3/1
  Zero-Order Hold17/1 -> P_loop/2(qd_des)
  pos5/1 -> S-Function24/1  "actuastatus5"
  Zero-Order Hold13/1 -> V_loop/1(V_in), V_out/1
  Data Type Conversion4/1 -> pos4/1
  Compare To Zero/1 -> Logical Operator12/2
  JOINT3 Average1/1 -> Mux4/6
  JOINT2 Average1/1 -> Mux4/2
  Saturation3/1 -> Product1/2
  Zero-Order Hold6/1 -> Mux2/6
  P_loop/2(err_too_big_flag) -> err/1
  JOINT3 Average/1 -> Mux4/3
  Data Type Conversion17/1 -> S-Function9/1
  f_ext/1 -> MJ_TAU/4(f_ext)
  S-Function36/1 -> Mux1/1
  disturb_gain/1 -> Saturation4/1
  S-Function32/1 -> Mux1/4
  G_correct_gain/1 -> Zero-Order Hold25/1, Add2/2, G/1
  Constant15/1 -> Switch8/1
  [joints_enable] -> Memory/1
  Logical Operator5/1 -> Logical Operator6/1
  tau_disturb/1 -> Scope11/1
  Constant13/1 -> Switch6/3
  Constant2/1 -> Saturation1/1
  Gain14/1 -> Zero-Order Hold8/1  "Encode2"
  Demux2/2 -> JOINT2 Average1/1
  Logical Operator13/1 -> V_loop/4(reset_integer)
  Data Type Conversion10/1 -> Gain13/1
  S-Function10/1 -> Zero-Order Hold4/1
  P_loop/1(V_out) -> Zero-Order Hold13/1
  Constant17/1 -> Switch11/3
  joint2_inver_dir3/1 -> Mux1/2
  q_degree/1 -> Scope16/1  "q_degree"
  n_ext/1 -> MJ_TAU/5(n_ext)
  Data Type Conversion3/1 -> pos5/1
  Mux6/1 -> Product2/1, tau_disturb/1
  Constant7/1 -> Switch3/3
  Constant6/1 -> Switch2/3
  Kff_coef/1 -> Saturation3/1
  disturb_6/1 -> Mux6/6
  MJ_G_compen/1(G_tau) -> G_correct_gain/1  "G_correct_gain"
  Demux2/5 -> Mux4/5
  S-Function23/1 -> Data Type Conversion12/1
  Data Type Conversion9/1 -> Gain12/1
  Product3/1 -> Discrete-Time Integrator/1
  Data Type Conversion1/1 -> pos6/1
  qd_degree/1 -> Scope5/1  "qd_degree"
  Switch7/1 -> Switch5/1
  G_and_fric/1 -> Scope10/1  "G_and_fric"
  disturb_4/1 -> Mux6/4
  joint2_inver_dir4/1 -> Mux2/2
  offset_q/1 -> Sum2/2
  Zero-Order Hold19/1 -> P_loop/3(q_actual)
  Constant10/1 -> Gain/1
  Data Type Conversion16/1 -> S-Function14/1
  Product5/1 -> Logical Operator2/1, Logical Operator3/1, Logical Operator5/1, Logical Operator4/1, Logical Operator1/1, Logical Operator/1
  [qd_actual] -> MJ_TAU/2(qd), Difference/1
  S-Function35/1 -> joint2_inver_dir3/1
  MJ_V_compen/1(C_tau) -> Zero-Order Hold26/1, C_tau/1
  S-Function2/1 -> Zero-Order Hold5/1
  Constant22/1 -> Switch11/1
  disturb_2/1 -> Mux6/2
  Logical Operator6/1 -> Mux3/6, Switch6/2
  M*qdd+C+G/1 -> tau_all/1
  atual_tau_rod/1 -> [actual_tau]  "atual_tau_rod"
  Product/1 -> M*qdd/1
  qd_des_t/1 -> Scope14/1  "qd_des_t"
  Demux/6 -> Data Type Conversion1/1
  Product4/1 -> Logical Operator1/2
  pos2/1 -> S-Function27/1  "actuastatus2"
  disturb_3/1 -> Mux6/3
  Gain16/1 -> Zero-Order Hold7/1  "Encode1"
  Mux/1 -> inc2rad/1(inc)
  V_out/1 -> Scope2/1  "V_out"
  Difference/1 -> Divide1/1
  S-Function1/1 -> Zero-Order Hold6/1
  [q_actual] -> MJ_M_matic/1(q)
  q_des_t/1 -> Scope6/1  "q_des_t"
  Zero-Order Hold9/1 -> Mux/3
  start/1 -> Scope3/1
  [q_actual] -> Subsystem6/2(q_actual_rad)
  MJ_M_matic/1(M) -> Zero-Order Hold27/1, Product/1
  pos3/1 -> S-Function26/1  "actuastatus3"
  Divide1/1 -> qdd/1
  Saturation4/1 -> Product2/2
  Switch1/1 -> Data Type Conversion16/1
  S-Function33/1 -> Mux1/3
  Data Type Conversion2/1 -> Gain10/1
  Zero-Order Hold15/1 -> Sum/1, tau_out/1
  Memory1/1 -> MJ_Traj2/2(q_des)
  Zero-Order Hold1/1 -> Mux2/1
  S-Function34/1 -> Mux1/5
  get_tau/1 -> atual_tau/1, atual_raw_tau/1  "actual_raw_tau"
  S-Function31/1 -> Mux1/6
  Constant21/1 -> Switch7/3
  Zero-Order Hold10/1 -> Mux/4
  [q_actual] -> MJ_V_compen/1(q)
  Switch6/1 -> Switch/1
  Switch10/1 -> Switch2/1
  Mux3/1 -> [joints_enable]
  joint2_inver_dir2/1 -> Data Type Conversion6/1
  MJ_Traj2/3(qd_des_t) -> Radians to Degrees3/1
  Divide/1 -> Scope/1, Demux2/1
  Demux2/4 -> Mux4/4
  MJ_Traj2/2(q_des_t) -> Radians to Degrees1/1
  disturb_5/1 -> Mux6/5
  Logical Operator1/1 -> Logical Operator10/1
  [q_actual] -> MJ_G_compen/1(q_actual)
  S-Function13/1 -> Data Type Conversion2/1
  C_tau/1 -> C/1
  Demux2/1 -> Mux4/1
  [qd_des] -> Radians to Degrees4/1, Zero-Order Hold17/1
  Radians to Degrees3/1 -> qd_des_t/1
  Data Type Conversion6/1 -> pos2/1
  [qd_des] -> MJ_frict_compen1/1(qd)
  Constant/1 -> S-Function7/1, S-Function8/1, S-Function6/1, S-Function5/1, S-Function4/1, S-Function3/1
  Constant19/1 -> Switch9/3
  Logical Operator3/1 -> Logical Operator8/1
  Data Type Conversion19/1 -> S-Function18/1
  tau_out/1 -> Scope18/1  "tau_out"
  enable6/1 -> Product9/2  "enable_6"
  Logical Operator2/1 -> Logical Operator9/1
  Constant3/1 -> atual_tau/2
  Switch8/1 -> Switch4/1
  pos4/1 -> S-Function25/1  "actuastatus4"
  Product7/1 -> Logical Operator3/2
  Switch9/1 -> Switch3/1
  Constant14/1 -> Switch6/1
  Constant18/1 -> Switch10/3
  Switch/1 -> Data Type Conversion17/1
  Gain/1 -> Scope13/1
  Logical Operator/1 -> Logical Operator11/1
  Product8/1 -> Logical Operator4/2
  [joints_enable] -> Sum of Elements/1
  Constant23/1 -> Switch10/1
  Product2/1 -> Sum/2
  joint2_inver_dir1/1 -> Mux/2
  Add2/1 -> G_and_fric/1, [feedforward_tau]
  S-Function19/1 -> Data Type Conversion8/1
  Switch11/1 -> Switch1/1
  Data Type Conversion11/1 -> Gain14/1
  S-Function22/1 -> Data Type Conversion11/1
  Constant16/1 -> Switch7/1
  Product6/1 -> Logical Operator2/2
  S-Function20/1 -> Data Type Conversion9/1
  Data Type Conversion8/1 -> Gain11/1
  tau_ff/1 -> feed_forward_tau/1  "tau_ff"
  MJ_frict_compen1/1(fric_new) -> fri_gain/1  "fri_gain"
  Mux4/1 -> Scope8/1, Demux/1
  inc2rad1/1(rad) -> Radians to Degrees2/1, [qd_actual], qd_rad/1
  fri_gain/1 -> Zero-Order Hold24/1, Add2/1
  Enabled Subsystem1/1(Out1) -> Memory1/1
  Sum1/1 -> V_loop/8(qd_actual_error), Scope1/1  "qd_degree_error"
  Radians to Degrees4/1 -> V_out2/1
  Radians to Degrees5/1 -> V_out1/1
  V_out1/1 -> Scope19/1, Sum1/2  "qd_actual_degree"
  V_out2/1 -> Sum1/1
  sim_Step/1 -> Discrete-Time Integrator1/1, Product3/1
  [qd_actual] -> Zero-Order Hold/1, Radians to Degrees5/1
  Constant26/1 -> Sum11/2
  V_out3/1 -> Sum5/1
  Radians to Degrees7/1 -> V_out4/1
  Radians to Degrees6/1 -> V_out3/1
  Sum5/1 -> V_loop/7(q_actual_error), Scope20/1  "q_degree_error"
  V_out4/1 -> Sum5/2
  P_loop/3(q_rad_error) -> V_loop/5(q_error)
  Sine Wave Function/1 -> Sum3/1
  Sine Wave Function3/1 -> Sum6/1
  Sine Wave Function4/1 -> Sum7/1
  Product10/1 -> Logical Operator/2
  enable_all/1 -> Product5/2
  Discrete-Time Integrator1/1 -> V_loop/6(clock), dingshichufa/1(t)
  Constant33/1 -> Saturation7/1
  Saturation7/1 -> Divide2/2
  Difference1/1 -> Divide2/1
  Subsystem6/1(change_flag) -> Enabled Subsystem1/Enable
  Logical Operator12/1 -> MJ_Traj2/1(start_enable), start/1
  Saturation/1 -> Enabled Subsystem1/1(In1)
  q_des_degree/1 -> degree2rad/1
  Difference2/1 -> Divide3/1
  Saturation9/1 -> Divide3/2
  degree2rad2/1 -> Saturation6/1
  Constant1/1 -> Saturation9/1
  Divide3/1 -> degree2rad2/1
  Saturation6/1 -> [qdd_des]
  [q_des] -> Zero-Order Hold18/1
  [qd_des] -> Zero-Order Hold20/1
  [qdd_des] -> Zero-Order Hold21/1
  [q_actual] -> Zero-Order Hold23/1
  Zero-Order Hold18/1 -> Sum4/2, Scope26/1
  Zero-Order Hold22/1 -> Sum8/1
  Sum8/1 -> 1dof_controller/2(x2), controller1/2(x2)
  Sum4/1 -> 1dof_controller/1(x1), fuzzy_logic_system6/1(x), fuzzy_logic_system5/1(x), fuzzy_logic_system4/1(x), fuzzy_logic_system3/1(x), fuzzy_logic_system2/1(x), fuzzy_logic_system1/1(x), controller1/1(x1)
  Zero-Order Hold21/1 -> 1dof_controller/7(thetad_ddot), controller1/7(thetad_ddot)
  controller1/3(nz2) -> Scope21/1  "nz2"
  Mux5/1 -> Scope27/1, degree2rad3/1, Difference1/1
  enable3/1 -> Product6/2
  enable4/1 -> Product7/2
  enable5/1 -> Product8/2
  Product9/1 -> Logical Operator5/2
  enable1/1 -> Product10/2
  enable2/1 -> Product4/2
  [qd_actual] -> Zero-Order Hold22/1
  Zero-Order Hold23/1 -> Sum4/1
  Zero-Order Hold24/1 -> 1dof_controller/6(F), controller1/6(F)
  Zero-Order Hold25/1 -> 1dof_controller/5(G), controller1/5(G)
  Zero-Order Hold26/1 -> 1dof_controller/4(V), controller1/4(V)
  degree2rad3/1 -> Saturation8/1
  Saturation8/1 -> Scope29/1, [q_des]
  degree2rad1/1 -> Saturation5/1
  Saturation5/1 -> [qd_des]
  Zero-Order Hold14/1 -> V_loop/2(forward_feed_tau)
  Zero-Order Hold20/1 -> Sum8/2, Scope25/1
  fuzzy_logic_system1/1(f) -> Mux7/1
  Mux7/1 -> controller1/8(f), qdd1/1
  fuzzy_logic_system2/1(f) -> Mux7/2
  Constant27/1 -> Sum6/2
  controller1/1(u) -> Saturation10/1
  Saturation10/1 -> Scope23/1
  fuzzy_logic_system3/1(f) -> Mux7/3
  Constant29/1 -> Sum7/2
  qdd1/1 -> Scope22/1  "fout"
  Constant12/1 -> Sum9/2
  Sine Wave Function1/1 -> Sum9/1
  fuzzy_logic_system4/1(f) -> Mux7/4
  Zero-Order Hold27/1 -> 1dof_controller/3(M), controller1/3(M)
  Sine Wave Function2/1 -> Sum10/1
  Sine Wave Function5/1 -> Sum11/1
  Discrete-Time Integrator/1 -> Sine Wave Function1/1, Sine Wave Function2/1, Sine Wave Function5/1, controller1/9(t), Sine Wave Function4/1, Sine Wave Function3/1, Sine Wave Function/1
  fuzzy_logic_system5/1(f) -> Mux7/5
  fuzzy_logic_system6/1(f) -> Mux7/6
  Constant25/1 -> Sum10/2
  Divide2/1 -> degree2rad1/1, Difference2/1
  controller1/2(nz1) -> Scope28/1  "nz1"
  Constant11/1 -> Mux5/6, Mux5/3, Mux5/2, Mux5/4
  Constant30/1 -> Mux5/5
  1dof_controller/1(u) -> Mux8/1
  1dof_controller/2(z1) -> Scope30/1  "z1"
  1dof_controller/3(z2) -> Scope31/1  "z2"
  Mux8/1 -> Sum12/1
  Sum12/1 -> Zero-Order Hold15/1
  V_loop/1(tau) -> Scope24/1, PID_gain/1
  PID_gain/1 -> ?  "PID_gain"
  Constant28/1 -> Mux5/1, Sum3/2
